simulink model "CSEI_model"  (R2015a)
settings: Solver=ode45  StartTime=0.0  StopTime=simlen  RelTol=1e-3
values from neighbouring files (symbols this model uses):
  b = [0;0;0]    [script_backstepping.m]
  center_xy = [6;0]    [script_backstepping.m]
  D = [-X_u,0,0 ... (first row only)    [script_backstepping.m]
  eta0 = [p0(1);p0(2);psi0]    [script_backstepping.m]
  integrator_reset = 0    [script_backstepping.m]
  K1 = 1*diag([0.01,0.01,0.6])    [script_backstepping.m]
  K2 = 0.3*diag([20,1,2])    [script_backstepping.m]
  K2_np = diag([wc_np_2 wc_np_2 wc_np_2])    [script_backstepping.m]
  K3_np = 0*diag([1 1 1])    [script_backstepping.m]
  K4_np = K3_np/wc_np_2    [script_backstepping.m]
  M = [m-X_u_dot,0,0 ... (first row only)    [script_backstepping.m]
  M_inverse = inv(M)    [script_backstepping.m]
  mu = 0.02    [script_backstepping.m]
  pd_0 = [2;0]    [script_backstepping.m]
  pd_1 = [10;4]    [script_backstepping.m]
  psi0 = 0    [script_backstepping.m]
  radii_xy = [5;3]    [script_backstepping.m]
  U_max = 0.1    [script_backstepping.m]
libraries: simulink_extras x1
settings Model: Creator=Shiv Jeet rai  LastModifiedBy=shivjr
settings DataIOCC: SaveFormat=Dataset
settings HardwareCC: ProdBitPerPointer=64  ProdLargestAtomicFloat=Float  ProdIntDivRoundTo=Zero  ProdEndianess=LittleEndian  ProdWordSize=64  ProdLongLongMode=on  ProdHWDeviceType=Intel->x86-64 (Windows64)
settings GRTTargetCC: GeneratePreprocessorConditionals=Use local settings
settings ConfigComp: CovMetricSettings=dw  CovHtmlReporting=on  CovSaveCumulativeToWorkspaceVar=on  CovSaveSingleToWorkspaceVar=on  CovExternalEMLEnable=off

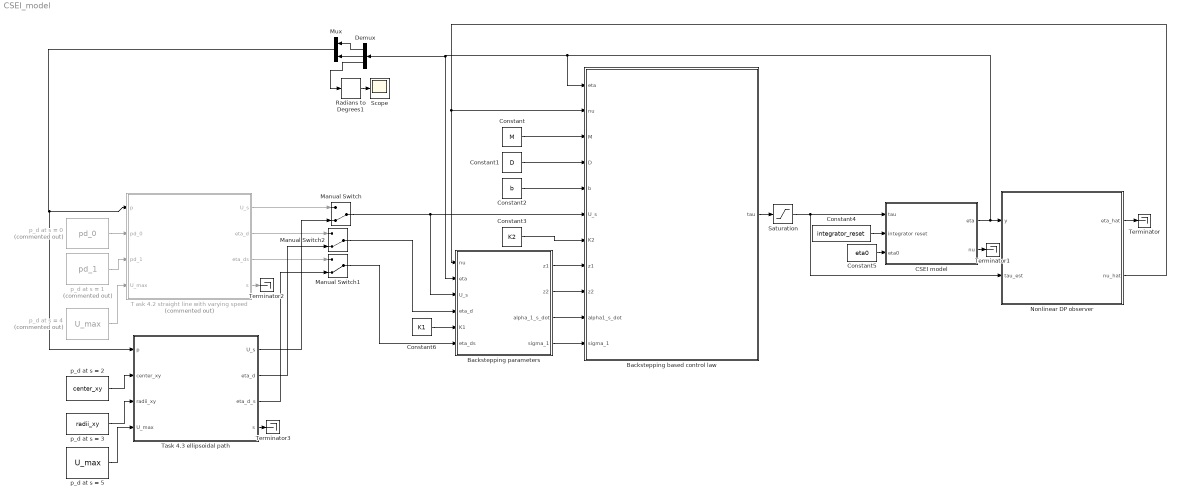
== system CSEI_model ==
  Backstepping based control law : MATLAB Function  TreatAsAtomicUnit=on
  Backstepping parameters : Subsystem
  CSEI model : Subsystem
  Constant : Constant  Value=M
  Constant1 : Constant  Value=D
  Constant2 : Constant  Value=b
  Constant3 : Constant  Value=K2
  Constant4 : Constant  Value=integrator_reset
  Constant5 : Constant  Value=eta0
  Constant6 : Constant  Value=K1
  Demux : Demux  Outputs=3
  Manual Switch : ManualSwitch  CurrentSetting=0
  Manual Switch1 : ManualSwitch  CurrentSetting=0
  Manual Switch2 : ManualSwitch  CurrentSetting=0
  Mux : Mux  Inputs=2
  Nonlinear DP observer : Subsystem
      settings: MinAlgLoopOccurrences=on
  Radians to Degrees1 : simulink_extras/Transformations/Radians to Degrees
  Saturation : Saturate  UpperLimit=[1.03;2.5;0.98]  LowerLimit=[-1.03;-2.5;-0.98]
  Scope : Scope
      settings: YMin=-0.06968  YMax=0.62714
  T ask 4.2 straight line with varying speed : Subsystem  Commented=on
  Task 4.3 ellipsoidal path : Subsystem
  Terminator{,1..3} (4 alike) : Terminator
  p_d at s = 0 : Constant  Commented=on  Value=pd_0
  p_d at s = 1 : Constant  Commented=on  Value=pd_1
  p_d at s = 2 : Constant  Value=center_xy
  p_d at s = 3 : Constant  Value=radii_xy
  p_d at s = 4 : Constant  Commented=on  Value=U_max
  p_d at s = 5 : Constant  Value=U_max
  wires:
  Backstepping parameters/1(z1) -> Backstepping based control law/8(z1)
  Backstepping parameters/2(z2) -> Backstepping based control law/9(z2)
  Backstepping parameters/3(alpha_1_s_dot) -> Backstepping based control law/10(alpha1_s_dot)
  Backstepping parameters/4(sigma_1) -> Backstepping based control law/11(sigma_1)
  Constant/1 -> Backstepping based control law/3(M)
  Constant1/1 -> Backstepping based control law/4(D)
  Constant2/1 -> Backstepping based control law/5(b)
  Constant3/1 -> Backstepping based control law/7(K2)
  Constant4/1 -> CSEI model/2(integrator reset)
  Constant5/1 -> CSEI model/3(eta0)
  Constant6/1 -> Backstepping parameters/5(K1)
  Mux/1 -> Task 4.3 ellipsoidal path/1(p), T ask 4.2 straight line with varying speed/1(p)
  Demux/1 -> Mux/1
  Demux/2 -> Mux/2
  Demux/3 -> Radians to Degrees1/1
  Backstepping based control law/1(tau) -> Saturation/1
  CSEI model/1(eta) -> Backstepping based control law/1(eta), Backstepping parameters/2(eta), Demux/1, Nonlinear DP observer/1(y)
  Radians to Degrees1/1 -> Scope/1
  p_d at s = 1/1 -> T ask 4.2 straight line with varying speed/3(pd_1)
  p_d at s = 0/1 -> T ask 4.2 straight line with varying speed/2(pd_0)
  Nonlinear DP observer/2(nu_hat) -> Backstepping based control law/2(nu), Backstepping parameters/1("nu ")
  Nonlinear DP observer/1(eta_hat) -> Terminator/1
  T ask 4.2 straight line with varying speed/1(U_s) -> Manual Switch/1
  T ask 4.2 straight line with varying speed/2(eta_d) -> Manual Switch2/1
  T ask 4.2 straight line with varying speed/3(eta_ds) -> Manual Switch1/1
  Manual Switch1/1 -> Backstepping parameters/6(eta_ds)
  Manual Switch2/1 -> Backstepping parameters/4(eta_d)
  Manual Switch/1 -> Backstepping parameters/3(U_s), Backstepping based control law/6(U_s)
  CSEI model/2(nu) -> Terminator1/1
  T ask 4.2 straight line with varying speed/4(s) -> Terminator2/1
  Task 4.3 ellipsoidal path/1(U_s) -> Manual Switch/2
  Task 4.3 ellipsoidal path/2(eta_d) -> Manual Switch2/2
  Task 4.3 ellipsoidal path/3(eta_d_s) -> Manual Switch1/2
  Task 4.3 ellipsoidal path/4("s ") -> Terminator3/1
  p_d at s = 3/1 -> Task 4.3 ellipsoidal path/3(radii_xy)
  p_d at s = 2/1 -> Task 4.3 ellipsoidal path/2(center_xy)
  Saturation/1 -> CSEI model/1(tau), Nonlinear DP observer/2("tau_est ")
  p_d at s = 4/1 -> T ask 4.2 straight line with varying speed/4(U_max)
  p_d at s = 5/1 -> Task 4.3 ellipsoidal path/4(U_max)

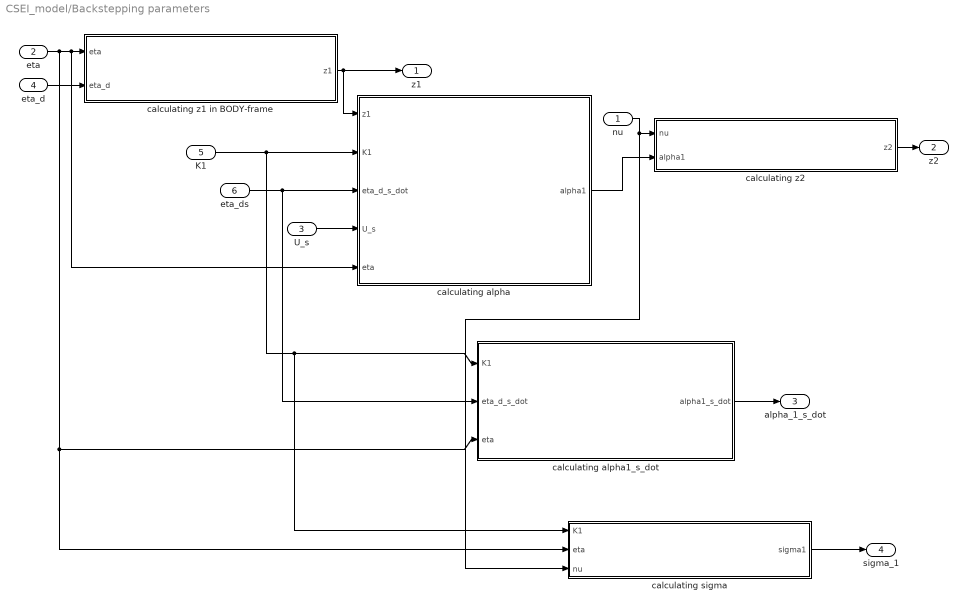
== system CSEI_model/Backstepping parameters ==
  "nu " : Inport
  eta : Inport  Port=2
  U_s : Inport  Port=3
  eta_d : Inport  Port=4
  K1 : Inport  Port=5
  eta_ds : Inport  Port=6
  calculating alpha : MATLAB Function  TreatAsAtomicUnit=on
  calculating alpha1_s_dot : MATLAB Function  TreatAsAtomicUnit=on
  "calculating sigma " : MATLAB Function  TreatAsAtomicUnit=on
  calculating z1 in BODY-frame : MATLAB Function  TreatAsAtomicUnit=on
  calculating z2 : MATLAB Function  TreatAsAtomicUnit=on
  z1 : Outport
  z2 : Outport  Port=2
  alpha_1_s_dot : Outport  Port=3
  sigma_1 : Outport  Port=4
  wires:
  calculating z1 in BODY-frame/1(z1) -> calculating alpha/1(z1), z1/1
  calculating z2/1(z2) -> z2/1
  "nu "/1 -> "calculating sigma "/3(nu), calculating z2/1(nu)
  eta_d/1 -> calculating z1 in BODY-frame/2(eta_d)
  calculating alpha/1(alpha1) -> calculating z2/2(alpha1)
  eta_ds/1 -> calculating alpha1_s_dot/2(eta_d_s_dot), calculating alpha/3(eta_d_s_dot)
  U_s/1 -> calculating alpha/4(U_s)
  calculating alpha1_s_dot/1(alpha1_s_dot) -> alpha_1_s_dot/1
  "calculating sigma "/1(sigma1) -> sigma_1/1
  K1/1 -> "calculating sigma "/1(K1), calculating alpha1_s_dot/1(K1), calculating alpha/2(K1)
  eta/1 -> "calculating sigma "/2(eta), calculating alpha1_s_dot/3(eta), calculating alpha/5(eta), calculating z1 in BODY-frame/1(eta)

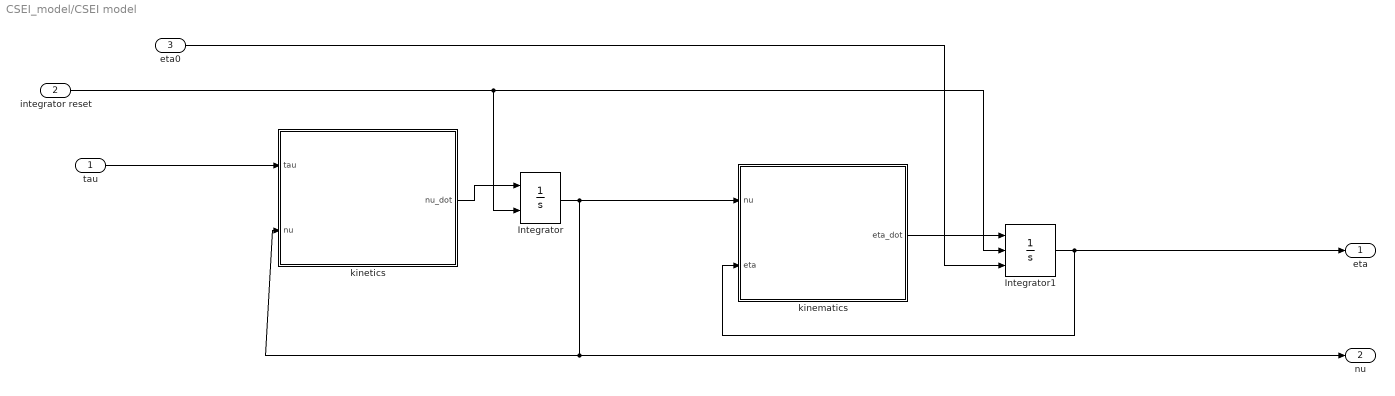
== system CSEI_model/CSEI model ==
  tau : Inport
  integrator reset : Inport  Port=2
  eta0 : Inport  Port=3
  Integrator : Integrator  ExternalReset=rising  InitialCondition=[0 0 0]'
  Integrator1 : Integrator  ExternalReset=rising  InitialConditionSource=external  InitialCondition=[0 0 0]'
  kinematics : MATLAB Function  TreatAsAtomicUnit=on
  kinetics : MATLAB Function  TreatAsAtomicUnit=on
  eta : Outport
  nu : Outport  Port=2
  wires:
  kinematics/1(eta_dot) -> Integrator1/1
  Integrator/1 -> nu/1, kinetics/2(nu), kinematics/1(nu)
  eta0/1 -> Integrator1/3
  kinetics/1(nu_dot) -> Integrator/1
  Integrator1/1 -> eta/1, kinematics/2(eta)
  tau/1 -> kinetics/1(tau)
  integrator reset/1 -> Integrator1/2, Integrator/2

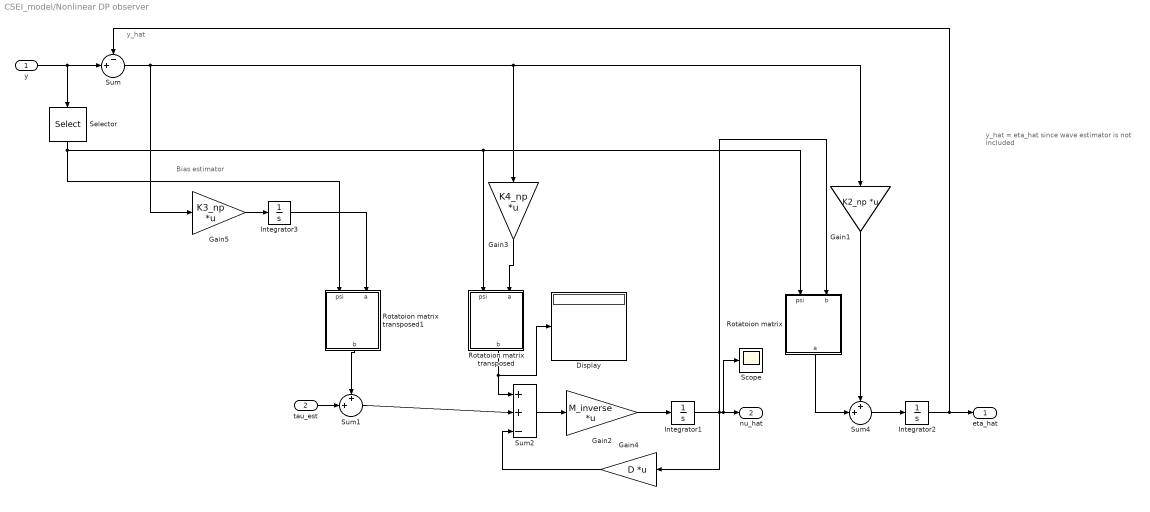
== system CSEI_model/Nonlinear DP observer ==
  note: y_hat
  note: y_hat = eta_hat
      | since wave estimator is not included
  note: Bias estimator
  y : Inport
  "tau_est " : Inport  Port=2
  Display : Display
  Gain1 : Gain  Gain=K2_np  Multiplication=Matrix(K*u)
  Gain2 : Gain  Gain=M_inverse  Multiplication=Matrix(K*u)
  Gain3 : Gain  Gain=K4_np  Multiplication=Matrix(K*u)
  Gain4 : Gain  Gain=D  Multiplication=Matrix(K*u)
  Gain5 : Gain  Gain=K3_np  Multiplication=Matrix(K*u)
  Integrator1 : Integrator
  Integrator2 : Integrator  InitialCondition=eta0
  Integrator3 : Integrator
  "Rotatoion matrix " : MATLAB Function  TreatAsAtomicUnit=on
  Rotatoion matrix transposed : MATLAB Function  TreatAsAtomicUnit=on
  Rotatoion matrix transposed1 : MATLAB Function  TreatAsAtomicUnit=on
  Scope : Scope
      settings: YMin=-0.04488  YMax=0.40392
  Selector : Selector  InputPortWidth=3  Indices=[3]
  Sum : Sum  Inputs=-+|
  Sum1 : Sum  Inputs=++|
  Sum2 : Sum  Inputs=++-|
  Sum4 : Sum  Inputs=++|
  eta_hat : Outport
  nu_hat : Outport  Port=2
  wires:
  y/1 -> Selector/1, Sum/2
  Gain3/1 -> Rotatoion matrix transposed/2(a)
  Sum1/1 -> Sum2/2
  Sum2/1 -> Gain2/1
  Gain2/1 -> Integrator1/1
  Gain4/1 -> Sum2/3
  Integrator1/1 -> "Rotatoion matrix "/2(b), Gain4/1, Scope/1, nu_hat/1
  Gain1/1 -> Sum4/1
  "Rotatoion matrix "/1(a) -> Sum4/2
  Sum4/1 -> Integrator2/1
  Integrator2/1 -> eta_hat/1, Sum/1
  "tau_est "/1 -> Sum1/2
  Sum/1 -> Gain5/1, Gain1/1, Gain3/1
  Rotatoion matrix transposed1/1(b) -> Sum1/1
  Selector/1 -> Rotatoion matrix transposed1/1(psi), "Rotatoion matrix "/1(psi), Rotatoion matrix transposed/1(psi)
  Rotatoion matrix transposed/1(b) -> Display/1, Sum2/1
  Integrator3/1 -> Rotatoion matrix transposed1/2(a)
  Gain5/1 -> Integrator3/1

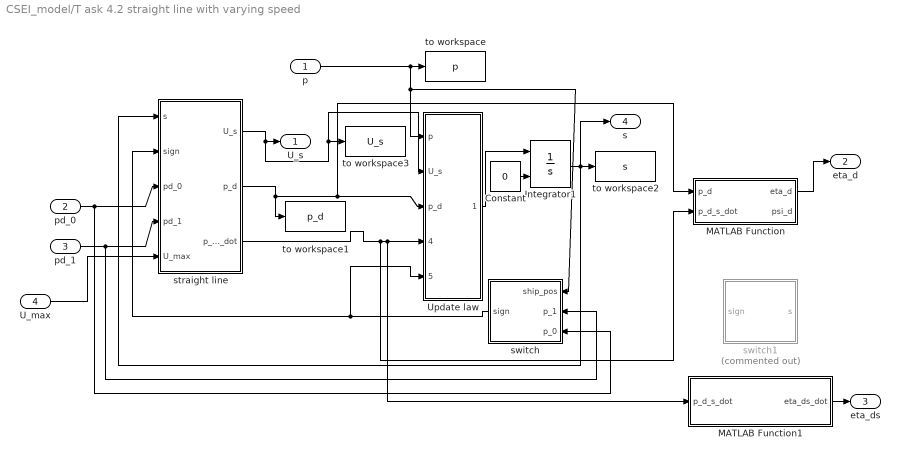
== system CSEI_model/T ask 4.2 straight line with varying speed ==
  p : Inport
  pd_0 : Inport  Port=2
  pd_1 : Inport  Port=3
  U_max : Inport  Port=4
  Constant : Constant  Value=0
  Integrator1 : Integrator  InitialConditionSource=external
  MATLAB Function : MATLAB Function  TreatAsAtomicUnit=on
  MATLAB Function1 : MATLAB Function  TreatAsAtomicUnit=on
  Update law : Subsystem
  straight line : Subsystem
  switch : Subsystem
  switch1 : Subsystem  Commented=on
  to workspace : ToWorkspace  VariableName=p  SaveFormat=Timeseries  SampleTime=-1
  to workspace1 : ToWorkspace  VariableName=p_d  SaveFormat=Timeseries  SampleTime=-1
  to workspace2 : ToWorkspace  VariableName=s  SaveFormat=Timeseries  SampleTime=-1
  to workspace3 : ToWorkspace  VariableName=U_s  SaveFormat=Timeseries  SampleTime=-1
  U_s : Outport
  eta_d : Outport  Port=2
  eta_ds : Outport  Port=3
  s : Outport  Port=4
  wires:
  Update law/1(s_dot) -> Integrator1/1
  switch/1(sign) -> Update law/5(sigma), straight line/2(sign)
  straight line/3(p_d_s_dot) -> MATLAB Function/2(p_d_s_dot), MATLAB Function1/1(p_d_s_dot), Update law/4(p_d_s_dot)
  Constant/1 -> Integrator1/2
  straight line/2(p_d) -> to workspace1/1, Update law/3(p_d), MATLAB Function/1(p_d)
  straight line/1(U_s) -> to workspace3/1, Update law/2(U_s), U_s/1
  Integrator1/1 -> s/1, to workspace2/1, straight line/1(s)
  p/1 -> switch/1(ship_pos), Update law/1(p), to workspace/1
  pd_0/1 -> switch/3(p_0), straight line/3(pd_0)
  pd_1/1 -> switch/2(p_1), straight line/4(pd_1)
  MATLAB Function/1(eta_d) -> eta_d/1
  MATLAB Function1/1(eta_ds_dot) -> eta_ds/1
  U_max/1 -> straight line/5(U_max)

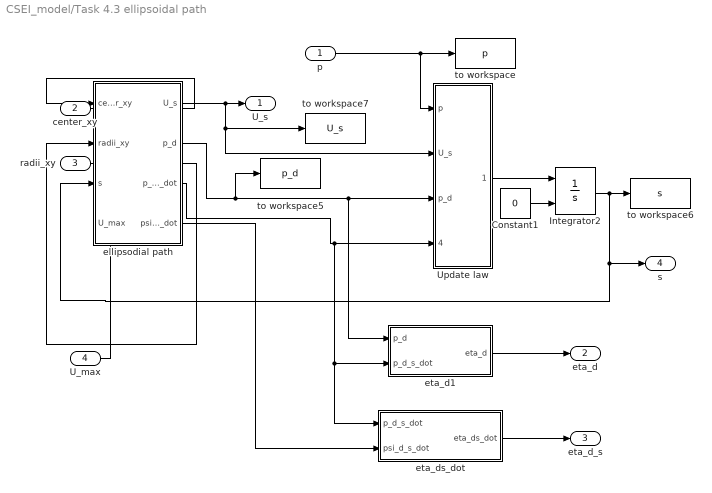
== system CSEI_model/Task 4.3 ellipsoidal path ==
  p : Inport
  center_xy : Inport  Port=2
  radii_xy : Inport  Port=3
  U_max : Inport  Port=4
  Constant1 : Constant  Value=0
  Integrator2 : Integrator  InitialConditionSource=external
  Update law : Subsystem
  ellipsodial path : Subsystem
  eta_d1 : Subsystem
  eta_ds_dot : MATLAB Function  TreatAsAtomicUnit=on
  to workspace : ToWorkspace  VariableName=p  SaveFormat=Timeseries  SampleTime=-1
  to workspace5 : ToWorkspace  VariableName=p_d  SaveFormat=Timeseries  SampleTime=-1
  to workspace6 : ToWorkspace  VariableName=s  SaveFormat=Timeseries  SampleTime=-1
  to workspace7 : ToWorkspace  VariableName=U_s  SaveFormat=Timeseries  SampleTime=-1
  U_s : Outport
  eta_d : Outport  Port=2
  eta_d_s : Outport  Port=3
  "s " : Outport  Port=4
  wires:
  p/1 -> Update law/1(p), to workspace/1
  Update law/1(s_dot) -> Integrator2/1
  ellipsodial path/3(p_d_s_dot) -> eta_ds_dot/1(p_d_s_dot), eta_d1/2(p_d_s_dot), Update law/4(p_d_s_dot)
  Constant1/1 -> Integrator2/2
  ellipsodial path/2(p_d) -> to workspace5/1, eta_d1/1(p_d), Update law/3(p_d)
  ellipsodial path/1(U_s) -> Update law/2(U_s), to workspace7/1, U_s/1
  Integrator2/1 -> ellipsodial path/3(s), "s "/1, to workspace6/1
  ellipsodial path/4(psi_d_s_dot) -> eta_ds_dot/2(psi_d_s_dot)
  center_xy/1 -> ellipsodial path/1(center_xy)
  radii_xy/1 -> ellipsodial path/2(radii_xy)
  eta_d1/1("eta_d ") -> eta_d/1
  eta_ds_dot/1(eta_ds_dot) -> eta_d_s/1
  U_max/1 -> ellipsodial path/4(U_max)

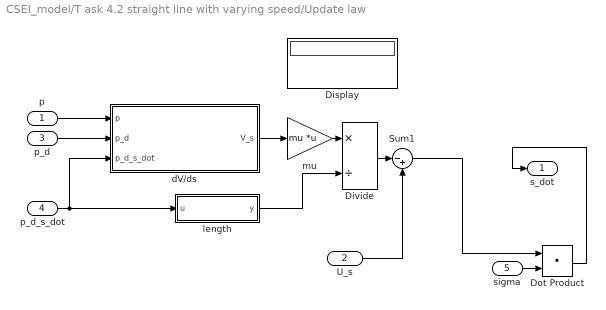
== system CSEI_model/T ask 4.2 straight line with varying speed/Update law ==
  p : Inport
  U_s : Inport  Port=2
  p_d : Inport  Port=3
  p_d_s_dot : Inport  Port=4
  sigma : Inport  Port=5
  Display : Display
  Divide : Product  Inputs=*/
  Dot Product : DotProduct  InputSameDT=on  OutDataTypeStr=Inherit: Inherit via internal rule
  Sum1 : Sum  Inputs=|-+
  "dV/ds  " : MATLAB Function  TreatAsAtomicUnit=on
  length : MATLAB Function  TreatAsAtomicUnit=on
  mu : Gain  Gain=mu  Multiplication=Matrix(K*u)
  s_dot : Outport
  wires:
  p/1 -> "dV/ds  "/1(p)
  mu/1 -> Divide/1
  Divide/1 -> Sum1/1
  "dV/ds  "/1(V_s) -> mu/1
  p_d/1 -> "dV/ds  "/2(p_d)
  p_d_s_dot/1 -> "dV/ds  "/3(p_d_s_dot), length/1(u)
  length/1(y) -> Divide/2
  Sum1/1 -> Dot Product/1
  Dot Product/1 -> s_dot/1
  sigma/1 -> Dot Product/2
  U_s/1 -> Sum1/2

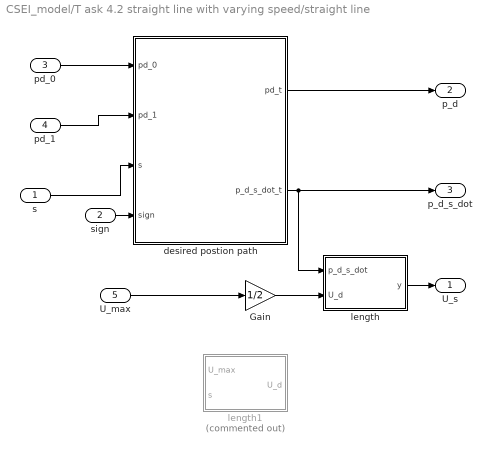
== system CSEI_model/T ask 4.2 straight line with varying speed/straight line ==
  s : Inport
  sign : Inport  Port=2
  pd_0 : Inport  Port=3
  pd_1 : Inport  Port=4
  U_max : Inport  Port=5
  Gain : Gain  Gain=1/2
  desired postion path : MATLAB Function  TreatAsAtomicUnit=on
  length : MATLAB Function  TreatAsAtomicUnit=on
  length1 : MATLAB Function  Commented=on  TreatAsAtomicUnit=on
  U_s : Outport
  p_d : Outport  Port=2
  p_d_s_dot : Outport  Port=3
  wires:
  desired postion path/1(pd_t) -> p_d/1
  desired postion path/2(p_d_s_dot_t) -> length/1(p_d_s_dot), p_d_s_dot/1
  length/1(y) -> U_s/1
  s/1 -> desired postion path/3(s)
  sign/1 -> desired postion path/4(sign)
  U_max/1 -> Gain/1
  pd_0/1 -> desired postion path/1(pd_0)
  pd_1/1 -> desired postion path/2(pd_1)
  Gain/1 -> length/2(U_d)

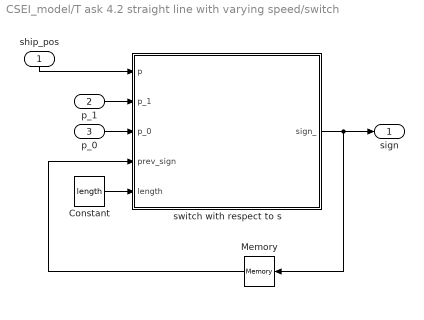
== system CSEI_model/T ask 4.2 straight line with varying speed/switch ==
  ship_pos : Inport
  p_1 : Inport  Port=2
  p_0 : Inport  Port=3
  Constant : Constant  Value=length
  Memory : Memory  X0=1
  switch with respect to s : MATLAB Function  TreatAsAtomicUnit=on
  sign : Outport
  wires:
  switch with respect to s/1(sign_) -> Memory/1, sign/1
  Memory/1 -> switch with respect to s/4(prev_sign)
  p_1/1 -> switch with respect to s/2(p_1)
  p_0/1 -> switch with respect to s/3(p_0)
  ship_pos/1 -> switch with respect to s/1(p)
  Constant/1 -> switch with respect to s/5(length)

== system CSEI_model/T ask 4.2 straight line with varying speed/switch1 ==
  s : Inport  PortDimensions=1
  Memory : Memory  X0=1
  switch with respect to s : MATLAB Function  TreatAsAtomicUnit=on
  sign : Outport
  wires:
  switch with respect to s/1(sign_) -> Memory/1, sign/1
  Memory/1 -> switch with respect to s/1(prev_sign)
  s/1 -> switch with respect to s/2(s)

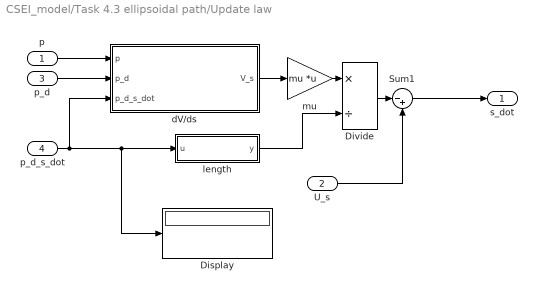
== system CSEI_model/Task 4.3 ellipsoidal path/Update law ==
  p : Inport
  U_s : Inport  Port=2
  p_d : Inport  Port=3
  p_d_s_dot : Inport  Port=4
  Display : Display
  Divide : Product  Inputs=*/
  Sum1 : Sum  Inputs=|-+
  "dV/ds  " : MATLAB Function  TreatAsAtomicUnit=on
  length : MATLAB Function  TreatAsAtomicUnit=on
  mu : Gain  Gain=mu  Multiplication=Matrix(K*u)
  s_dot : Outport
  wires:
  p/1 -> "dV/ds  "/1(p)
  mu/1 -> Divide/1
  Divide/1 -> Sum1/1
  "dV/ds  "/1(V_s) -> mu/1
  p_d/1 -> "dV/ds  "/2(p_d)
  p_d_s_dot/1 -> "dV/ds  "/3(p_d_s_dot), Display/1, length/1(u)
  length/1(y) -> Divide/2
  U_s/1 -> Sum1/2
  Sum1/1 -> s_dot/1

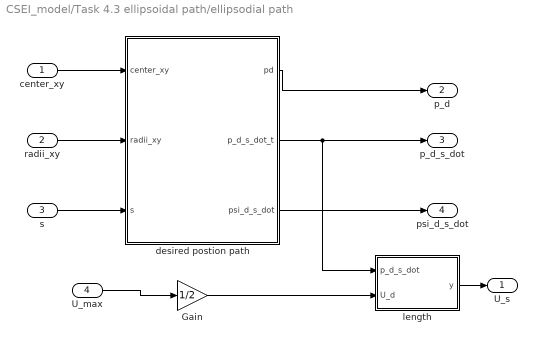
== system CSEI_model/Task 4.3 ellipsoidal path/ellipsodial path ==
  center_xy : Inport
  radii_xy : Inport  Port=2
  s : Inport  Port=3
  U_max : Inport  Port=4
  Gain : Gain  Gain=1/2
  desired postion path : MATLAB Function  TreatAsAtomicUnit=on
  length : MATLAB Function  TreatAsAtomicUnit=on
  U_s : Outport
  p_d : Outport  Port=2
  p_d_s_dot : Outport  Port=3
  psi_d_s_dot : Outport  Port=4
  wires:
  desired postion path/1(pd) -> p_d/1
  desired postion path/2(p_d_s_dot_t) -> length/1(p_d_s_dot), p_d_s_dot/1
  length/1(y) -> U_s/1
  s/1 -> desired postion path/3(s)
  desired postion path/3(psi_d_s_dot) -> psi_d_s_dot/1
  center_xy/1 -> desired postion path/1(center_xy)
  radii_xy/1 -> desired postion path/2(radii_xy)
  Gain/1 -> length/2(U_d)
  U_max/1 -> Gain/1

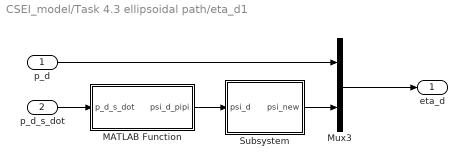
== system CSEI_model/Task 4.3 ellipsoidal path/eta_d1 ==
  p_d : Inport
  p_d_s_dot : Inport  Port=2
  MATLAB Function : MATLAB Function  TreatAsAtomicUnit=on
  Mux3 : Mux  Inputs=2
  Subsystem : Subsystem
  "eta_d " : Outport
  wires:
  Subsystem/1(psi_new) -> Mux3/2
  Mux3/1 -> "eta_d "/1
  MATLAB Function/1(psi_d_pipi) -> Subsystem/1(psi_d)
  p_d/1 -> Mux3/1
  p_d_s_dot/1 -> MATLAB Function/1(p_d_s_dot)

== system CSEI_model/Task 4.3 ellipsoidal path/eta_d1/Subsystem ==
  psi_d : Inport
  Delay : Delay  DelayLength=1  InitialCondition=psi0  SampleTime=0.1
  Delay1 : Delay  DelayLength=1  InitialCondition=0  SampleTime=0.1
  MATLAB Function2 : MATLAB Function  TreatAsAtomicUnit=on
  Scope : Scope
      settings: YMin=-0.25  YMax=2.25  SaveName=ScopeData6
  psi_new : Outport
  wires:
  MATLAB Function2/1(psi_new) -> psi_new/1
  psi_d/1 -> Delay/1, MATLAB Function2/1(psi_d)
  Delay1/1 -> MATLAB Function2/3(counter)
  Delay/1 -> MATLAB Function2/2(psi_prev)
  MATLAB Function2/2(counter_out) -> Scope/1, Delay1/1

== matlab function CSEI_model/CSEI model/kinematics ==
  data: nu input; eta_dot output; eta input
function eta_dot = CSE1_eta_dot(nu,eta)

psi = eta(3);

J = [cos(psi) -sin(psi) 0
     sin(psi) cos(psi)  0
     0        0         1];

eta_dot = J*nu;

== matlab function CSEI_model/CSEI model/kinetics ==
  data: tau input; nu_dot output; nu input
function nu_dot = CSE1_nu_dot(tau,nu)

u   = nu(1);
v   = nu(2);
r   = nu(3);

tau = [tau(1);tau(2);tau(3)];
%% MATRICES

m    = 14.79;   I_z  =  1.7600;   x_g = 0.0375;       % x_g  =  0.0460; % Table B.1


%% Added mass
X_ud  =     -2.0;											% Table B.1
					Y_vd =     -1.0;	N_vd =    -0.0;		% Table B.1 guestimate
					Y_rd =      -0.0;	N_rd =    -1.0;		% Table B.1

%% Total mass matrix
m_11 = m-X_ud;
m_22 = m-Y_vd;
m_23 = m*x_g-Y_rd;
m_32 = m*x_g-N_vd;
m_33 = I_z-N_rd;

M    = [m_11 0    0
        0    m_22 m_23
        0    m_32 m_33];
	
%% Damping coefficients
% Comments at the end of the lines indicate the old values used.
X_u		= -0.6555;		X_v		= 0;
X_uu 	= 0.3545;		X_vv	= -2.443;
X_uuu 	= -3.787;		X_vvv	= 0;

						Y_v		= -1.33; 			Y_r		= -7.250; % Y_r
						Y_vv	= -2.776;			Y_rr	= -3.450; % Y_rr
						Y_vvv	= -64.91;			Y_rrr	= 0;
						
						Y_rv	= -0.805;			Y_vr	= -0.845; % Y_rv, Y_vr

						N_v		= 0;				N_r		= -1.900; % N_r
						N_vv	= -0.2088;			N_rr	= -0.750; % N_rr
						N_vvv	= 0;				N_rrr	= 0;
						
						N_rv	= 0.130;			N_vr	= 0.080; % N_rv, N_vr

%% Correolis matrix
c_13 = -(m-Y_vd)*v-(m*x_g-Y_rd)*r;
c_23 = (m-X_ud)*u;
C    = [0     0     c_13
        0     0     c_23
        -c_13 -c_23 0   ];

%% Assembly of the damping matrix
d_11 = -X_u - X_uu*u - X_uuu*u^2;
d_22 = -Y_v - Y_vv*v - Y_vvv*v^2 - Y_rv*abs(r);
d_33 = -N_r - N_rr*abs(r) - N_rrr*r^2 - N_vr*abs(v); % using abs(r)

d_12 = -X_v - X_vv*v - X_vvv*v^2;
d_23 = -Y_r - Y_rr*abs(r) - Y_rrr*r^2 - Y_vr*abs(v);
d_32 = -N_v - N_vv*v - N_vvv*v^2 - N_rv*abs(r);

D    = [d_11 d_12 0
        0    d_22 d_23
        0    d_32 d_33];



%% CALCULATION
nu_dot = M\(tau-(C+D)*nu);

== matlab function CSEI_model/Backstepping based control law ==
  data: eta input; nu input; M input; D input; b input; U_s input; K2 input; z1 input; tau output; z2 input; alpha1_s_dot input; sigma_1 input size=[3 1]
function tau = fcn(eta, nu, M, D, b, U_s, K2, z1, z2, alpha1_s_dot,sigma_1)
%#codegen
psi = eta(3);
R = [   cos(psi)    -sin(psi)   0;
        sin(psi)    cos(psi)    0;
        0           0           1;];  
tau = -z1 + D*nu - transpose(R)*b + M*alpha1_s_dot*U_s + M*sigma_1 - K2*z2;

== matlab function CSEI_model/T ask 4.2 straight line with varying speed/Update law/length ==
  data: u input; y output
function y = fcn(u)

y = sqrt(u(1)^2 + u(2)^2);

== matlab function CSEI_model/T ask 4.2 straight line with varying speed/Update law/dV//ds   ==
  data: p input; V_s output; p_d input; p_d_s_dot input
function V_s = fcn(p, p_d, p_d_s_dot)

temp = - transpose(p - p_d)*p_d_s_dot;
V_s = temp;

== matlab function CSEI_model/T ask 4.2 straight line with varying speed/straight line/length1 ==
  data: U_max input; U_d output; s input
function U_d = fcn(U_max,s)

% if s > 1
%     s = 1;
% elseif s < 0
%     s = 0;
% end

U_d = U_max*(1.01 + sin(2*pi*s - pi/2));

== matlab function CSEI_model/Backstepping parameters/calculating alpha ==
  data: z1 input size=[3 1]; K1 input; alpha1 output; eta_d_s_dot input size=[3 1]; U_s input size=1; eta input size=[3 1]
function alpha1 = fcn(z1,K1, eta_d_s_dot, U_s, eta)
%#codegen
psi = eta(3);
R = [   cos(psi)    -sin(psi)   0;
        sin(psi)    cos(psi)    0;
        0           0           1;];  

alpha1 = -K1*z1 + transpose(R)*eta_d_s_dot*U_s;

== matlab function CSEI_model/T ask 4.2 straight line with varying speed/straight line/desired postion path ==
  data: pd_0 input; pd_1 input; pd_t output; p_d_s_dot_t output; s input size=1; sign input size=1
function [pd_t,p_d_s_dot_t] = fcn(pd_0,pd_1,s, sign)

if s >= 1
    s = 1;
elseif s <= 0
    s = 0;
end

p_d_s_dot_t = [ (pd_1(1)-pd_0(1));%*sign; 
                (pd_1(2)-pd_0(2))];%;*sign];

pd_t =  [(pd_1(1)-pd_0(1))*s + pd_0(1);
         (pd_1(2)-pd_0(2))*s + pd_0(2)];   
end

== matlab function CSEI_model/T ask 4.2 straight line with varying speed/straight line/length ==
  data: p_d_s_dot input; y output; U_d input
function y = fcn(p_d_s_dot,U_d)

y = U_d/sqrt(p_d_s_dot(1)^2 + p_d_s_dot(2)^2);

== matlab function CSEI_model/Backstepping parameters/calculating alpha1_s_dot ==
  data: K1 input size=[3 3]; eta_d_s_dot input size=[3 1]; alpha1_s_dot output size=[3 1]; eta input size=[3 1]
function alpha1_s_dot = fcn(K1, eta_d_s_dot, eta)
%#codegen
psi = eta(3);
R = [   cos(psi)    -sin(psi)   0;
        sin(psi)    cos(psi)    0;
        0           0           1;];  

alpha1_s_dot = K1*transpose(R)*eta_d_s_dot;

== matlab function CSEI_model/Backstepping parameters/calculating sigma  ==
  data: sigma1 output size=[3 1]; K1 input; eta input; nu input
function sigma1 = fcn(K1,eta,nu)
%Skew_symmetric_matrix =  
S = [0 -1 1;
     1 0 -1;
     -1 1 0;];

psi = eta(3);
R = [   cos(psi)    -sin(psi)   0;
        sin(psi)    cos(psi)    0;
        0           0           1;];

r = nu(3);
sigma1 = K1*S*eta*r - nu;

== matlab function CSEI_model/Backstepping parameters/calculating z1 in BODY-frame ==
  data: z1 output size=[3 1]; eta input size=[3 1]; eta_d input size=[3 1]
function z1 = fcn(eta, eta_d)
%#codegen
psi = eta(3);
R = [   cos(psi)    -sin(psi)   0;
        sin(psi)    cos(psi)    0;
        0           0           1;];  
z1 = transpose(R)*(eta-eta_d);

== matlab function CSEI_model/Backstepping parameters/calculating z2 ==
  data: z2 output size=[3 1]; nu input size=[3 1]; alpha1 input size=[3 1]
function z2 = fcn(nu, alpha1)
%#codegen

z2 = nu-alpha1;

== matlab function CSEI_model/T ask 4.2 straight line with varying speed/switch/switch with respect to s ==
  data: p input size=[2 1]; p_1 input size=[2 1]; p_0 input size=[2 1]; sign_ output size=1; prev_sign input size=1; length input size=1
function sign_  = fcn(p, p_1, p_0, prev_sign, length)

x_1 = (p(1) - p_1(1))^2; 
y_1 = (p(2) - p_1(2))^2;

x_0 = (p(1) - p_0(1))^2; 
y_0 = (p(2) - p_0(2))^2;

if length > sqrt(x_1^2 + y_1^2) %inside the acceptance area for point 1
    sign_ = -1;
elseif length > sqrt(x_0^2 + y_0^2)
        sign_ = 1;
else
    sign_ = prev_sign;
end

== matlab function CSEI_model/T ask 4.2 straight line with varying speed/MATLAB Function ==
  data: p_d input; p_d_s_dot input; eta_d output; psi_d output
function [eta_d,psi_d] = fcn(p_d,p_d_s_dot)
%#codegen
psi_d = atan2(p_d_s_dot(2),p_d_s_dot(1));

eta_d = [p_d(1); p_d(2); psi_d];

== matlab function CSEI_model/T ask 4.2 straight line with varying speed/MATLAB Function1 ==
  data: p_d_s_dot input; eta_ds_dot output
function eta_ds_dot = fcn(p_d_s_dot)
%#codegen
eta_ds_dot = [p_d_s_dot(1);p_d_s_dot(2);0];

== matlab function CSEI_model/Nonlinear DP observer/Rotatoion matrix transposed ==
  data: psi input; a input; b output
function b = fcn(psi, a)
%#codegen
R = [   cos(psi)    -sin(psi)   0;
        sin(psi)    cos(psi)    0;
        0           0           1;];  
b = transpose(R)*a;

== matlab function CSEI_model/Nonlinear DP observer/Rotatoion matrix transposed1 ==
  data: psi input; a input; b output
function b = fcn(psi, a)
%#codegen
R = [   cos(psi)    -sin(psi)   0;
        sin(psi)    cos(psi)    0;
        0           0           1;];  
b = transpose(R)*a;

== matlab function CSEI_model/Nonlinear DP observer/Rotatoion matrix  ==
  data: psi input; a output size=[3 1]; b input size=[3 1]
function a = fcn(psi, b)
%#codegen
R = [   cos(psi)    -sin(psi)   0;
        sin(psi)    cos(psi)    0;
        0           0           1;];  
a = R*b;

== matlab function CSEI_model/T ask 4.2 straight line with varying speed/switch1/switch with respect to s ==
  data: prev_sign input size=1; s input size=1; sign_ output size=1
function sign_  = fcn(prev_sign, s)

if s > 1
    sign_ = -1;
elseif s < 0
        sign_ = 1;
else
    sign_ = prev_sign;
end

== matlab function CSEI_model/Task 4.3 ellipsoidal path/Update law/dV//ds   ==
  data: p input; V_s output; p_d input; p_d_s_dot input
function V_s = fcn(p, p_d, p_d_s_dot)

temp = - transpose(p - p_d)*p_d_s_dot;
V_s = temp;

== matlab function CSEI_model/Task 4.3 ellipsoidal path/Update law/length ==
  data: u input; y output
function y = fcn(u)

y = sqrt(u(1)^2 + u(2)^2);

== matlab function CSEI_model/Task 4.3 ellipsoidal path/ellipsodial path/desired postion path ==
  data: center_xy input; radii_xy input; pd output; p_d_s_dot_t output; s input size=1; psi_d_s_dot output
function [pd,p_d_s_dot_t,psi_d_s_dot] = fcn(center_xy,radii_xy,s)

p_d_s_dot_t = [ -2*pi*radii_xy(1)*sin(2*pi*s); 
                2*pi*radii_xy(2)*cos(2*pi*s)];
            
p_d_s2 =  [ -(2*pi)^2*radii_xy(1)*cos(2*pi*s); 
                -(2*pi)^2*radii_xy(2)*sin(2*pi*s)];
            
psi_d_s_dot = (p_d_s_dot_t(1)*p_d_s2(2) - p_d_s2(1)*p_d_s_dot_t(2)) / (p_d_s_dot_t(1)^2 + p_d_s_dot_t(2)^2);

pd =  [ radii_xy(1)*cos(2*pi*s)+center_xy(1);
        radii_xy(2)*sin(2*pi*s)+center_xy(2)];   
end

== matlab function CSEI_model/Task 4.3 ellipsoidal path/ellipsodial path/length ==
  data: p_d_s_dot input; y output; U_d input
function y = fcn(p_d_s_dot,U_d)

y = U_d/sqrt(p_d_s_dot(1)^2 + p_d_s_dot(2)^2);

== matlab function CSEI_model/Task 4.3 ellipsoidal path/eta_d1/MATLAB Function ==
  data: p_d_s_dot input; psi_d_pipi output
function psi_d_pipi = fcn(p_d_s_dot)
%#codegen
psi_d_pipi = atan2(p_d_s_dot(2),p_d_s_dot(1));

== matlab function CSEI_model/Task 4.3 ellipsoidal path/eta_d1/Subsystem/MATLAB Function2 ==
  data: psi_d input; psi_new output; psi_prev input; counter input; counter_out output
function [psi_new,counter_out] = fcn(psi_d,psi_prev,counter)
%#codegen

if psi_d - psi_prev < -2*pi + 0.4 %Clockwise movement
    counter_out = counter + 1;
    %psi_new = psi_d + 2*pi*counter_out;
elseif psi_d - psi_prev > 2*pi - 0.4 %Counter clockwise movement
    counter_out = counter - 1;
    %psi_new = psi_d + 2*pi*counter_out;
else
    %psi_new = psi_d + 2*pi*counter;
    counter_out = counter;
end
psi_new = psi_d + 2*pi*counter_out;

== matlab function CSEI_model/Task 4.3 ellipsoidal path/eta_ds_dot ==
  data: p_d_s_dot input; eta_ds_dot output; psi_d_s_dot input
function eta_ds_dot = fcn(p_d_s_dot,psi_d_s_dot)
%#codegen
eta_ds_dot = [p_d_s_dot(1);p_d_s_dot(2);psi_d_s_dot];
